simulink model "Step_Response_t"  (Simulink 7.7)
settings: Solver=ode45  StartTime=0.0  StopTime=10  RelTol=1e-3
libraries: dspsnks4 x9
settings Model: Creator=Kaustubh C Shivdikar  LastModifiedBy=Kaustubh C Shivdikar

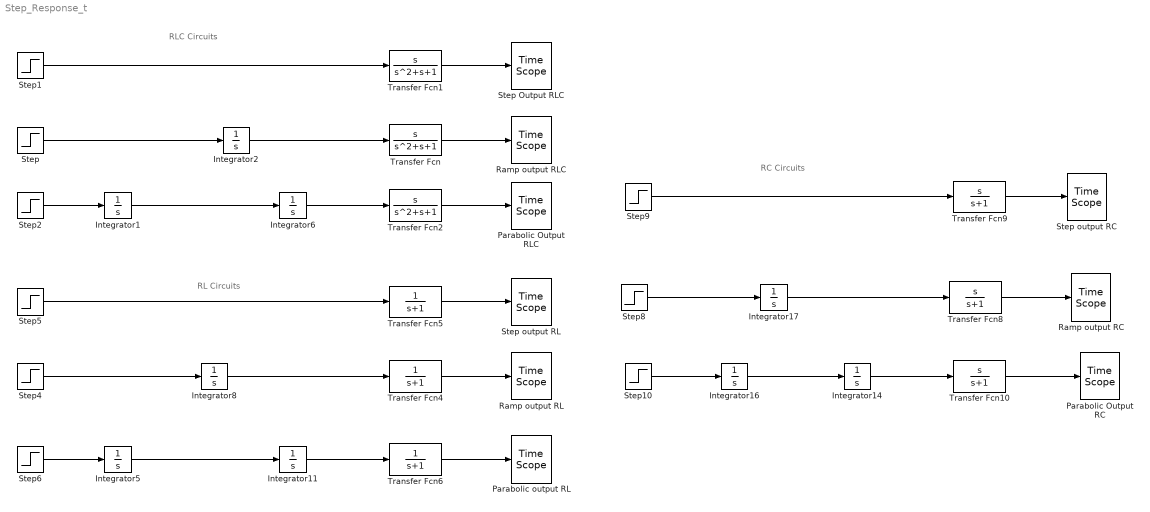
== system Step_Response_t ==
  note: RLC Circuits
  note: RL Circuits
  note: RC Circuits
  Integrator{1..2,5..6,8,11,14,16..17} (9 alike) : Integrator
  Parabolic Output RC : dspsnks4/Time Scope
  Parabolic Output RLC : dspsnks4/Time Scope
  Parabolic output RL : dspsnks4/Time Scope
  Ramp output RC : dspsnks4/Time Scope
  Ramp output RL : dspsnks4/Time Scope
  Ramp output RLC : dspsnks4/Time Scope
  Step{,1..2,4..6,8..10} (9 alike) : Step  Time=0  SampleTime=0
  "Step Output RLC " : dspsnks4/Time Scope
  Step output RC : dspsnks4/Time Scope
  Step output RL : dspsnks4/Time Scope
  Transfer Fcn : TransferFcn  Numerator=[1 0]  Denominator=[1 1 1]
  Transfer Fcn1 : TransferFcn  Numerator=[1 0]  Denominator=[1 1 1]
  Transfer Fcn10 : TransferFcn  Numerator=[1 0]  Denominator=[1 1]
  Transfer Fcn2 : TransferFcn  Numerator=[1 0]  Denominator=[1 1 1]
  Transfer Fcn4 : TransferFcn  Denominator=[1 1]
  Transfer Fcn5 : TransferFcn  Denominator=[1 1]
  Transfer Fcn6 : TransferFcn  Denominator=[1 1]
  Transfer Fcn8 : TransferFcn  Numerator=[1 0]  Denominator=[1 1]
  Transfer Fcn9 : TransferFcn  Numerator=[1 0]  Denominator=[1 1]
  wires:
  Transfer Fcn/1 -> Ramp output RLC/1
  Step1/1 -> Transfer Fcn1/1
  Transfer Fcn1/1 -> "Step Output RLC "/1
  Step/1 -> Integrator2/1
  Integrator2/1 -> Transfer Fcn/1
  Step2/1 -> Integrator1/1
  Integrator1/1 -> Integrator6/1
  Integrator6/1 -> Transfer Fcn2/1
  Step5/1 -> Transfer Fcn5/1
  Step4/1 -> Integrator8/1
  Integrator8/1 -> Transfer Fcn4/1
  Step6/1 -> Integrator5/1
  Integrator5/1 -> Integrator11/1
  Integrator11/1 -> Transfer Fcn6/1
  Step9/1 -> Transfer Fcn9/1
  Step8/1 -> Integrator17/1
  Integrator17/1 -> Transfer Fcn8/1
  Step10/1 -> Integrator16/1
  Integrator16/1 -> Integrator14/1
  Integrator14/1 -> Transfer Fcn10/1
  Transfer Fcn2/1 -> Parabolic Output RLC/1
  Transfer Fcn5/1 -> Step output RL/1
  Transfer Fcn4/1 -> Ramp output RL/1
  Transfer Fcn6/1 -> Parabolic output RL/1
  Transfer Fcn9/1 -> Step output RC/1
  Transfer Fcn8/1 -> Ramp output RC/1
  Transfer Fcn10/1 -> Parabolic Output RC/1
